simulink model "rfdc_V0_4"  (R2018a)
settings: Solver=VariableStepAuto  StartTime=0.0  StopTime=10.0  RelTol=1e-3
libraries: xbsIndex_r4 x2
settings Model: Creator=wei  LastModifiedBy=wei

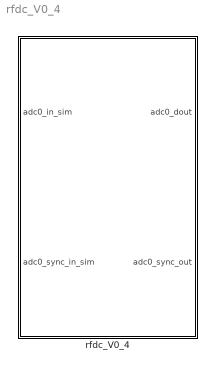
== system rfdc_V0_4 ==
  rfdc_V0_4 : Subsystem  Tag=xps:rfdc_V0_4  mask(rfdc){sys_config=1 ADC CORE, adc_sample_rate=2048, mts_mode=Non-MTS}
      mask prompts: sys_config "System Configuration"; adc_sample_rate "ADC Clock Rate(MHz)"; mts_mode "MTS Mode"
      mask help: This is for implementing RFDC core in RFSOC.
      mask init:
      | rfdc_v0_4_init(gcb,...
      |     'sys_config',sys_config,...
      |     'adc_sample_rate',adc_sample_rate,...
      |     'mts_mode',mts_mode);
      mask TypeOptions sys_config: 1 ADC CORE | 2 ADC CORES | 4 ADC CORES | 8 ADC CORES
      mask TypeOptions adc_sample_rate: 2048 | 4096
      mask TypeOptions mts_mode: Non-MTS | MTS

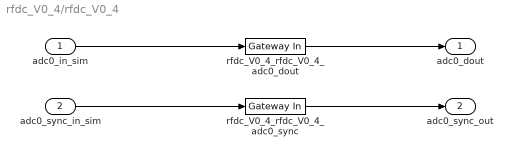
== system rfdc_V0_4/rfdc_V0_4 ==
  adc0_in_sim : Inport
  adc0_sync_in_sim : Inport  Port=2
  rfdc_V0_4_rfdc_V0_4_adc0_dout : xbsIndex_r4/Gateway In  gui_display_data_type=Fixed-point  arith_type=Unsigned  n_bits=128  bin_pt=0  preci_type=Single  exp_width=8  frac_width=24  rows=1  columns=1  quantization=Truncate  overflow=Wrap  period=1  UseAsADC=off  ADCChannel='1'  interface=None  automatic_assignment=on  address_offset=hex2dec('00')  intf_name=''  intf_description=''  default_value=0  timing_constraint=None  locs_specified=off  LOCs={}  io_standard={}  inherit_from_input=off  hdl_port=on  dbl_ovrd=off  block_type=gatewayin
  rfdc_V0_4_rfdc_V0_4_adc0_sync : xbsIndex_r4/Gateway In  gui_display_data_type=Fixed-point  arith_type=Boolean  n_bits=1  bin_pt=0  preci_type=Single  exp_width=8  frac_width=24  rows=1  columns=1  quantization=Truncate  overflow=Wrap  period=1  UseAsADC=off  ADCChannel='1'  interface=None  automatic_assignment=on  address_offset=hex2dec('00')  intf_name=''  intf_description=''  default_value=0  timing_constraint=None  locs_specified=off  LOCs={}  io_standard={}  inherit_from_input=off  hdl_port=on  dbl_ovrd=off  block_type=gatewayin
  adc0_dout : Outport
  adc0_sync_out : Outport  Port=2
  wires:
  adc0_in_sim/1 -> rfdc_V0_4_rfdc_V0_4_adc0_dout/1
  rfdc_V0_4_rfdc_V0_4_adc0_dout/1 -> adc0_dout/1
  adc0_sync_in_sim/1 -> rfdc_V0_4_rfdc_V0_4_adc0_sync/1
  rfdc_V0_4_rfdc_V0_4_adc0_sync/1 -> adc0_sync_out/1
